simulink model "Overtaking_Integrated"  (R2020b)
settings: Solver=ode23tb  StartTime=0.0  StopTime=25  FixedStep=.01  RelTol=5e-3  EnableMultiTasking=on
InitFcn:
  | %SimulationParameters;
StartFcn:
  | %tic
StopFcn:
  | %toc
  | save(['SimOutputs\' char(datetime('now','Format','y_M_d_HH_mm_ss')) '_' 'sim_out.mat'], 'logsout');
model workspace (MAT data in the model file):
  DLCXref = [-3.2158 4.0142 4.2842 14.7842 29.7842 30.2842 41.7842 46.7842 56.7842]
  DLCYref = [-3.1012 -3.1012 -7.6012 -7.1012 -6.8512 -1.6012 -1.8512 -3.1012 -3.1012]
  Downshift_Speeds = [9.5625  23.0625  36.5625  47.8125  59.0625  68.90625  78.75; 12.9375  26.4375  39.9375  51.1875  62.4375  72.84375  83.25; 16.3125  29.8125  43.3125  54.5625  65.8125  76.78125  87.75; 19.6875  33.1875  46.6875  57.9375  69.1875  80.71875  92.25]
  EngRevLim = 7000
  Pedal_Positions = [0.1 0.4 0.5 0.9]
  Upshift_Speeds = [12.9375  26.4375  39.9375  51.1875  62.4375  72.84375  83.25; 16.3125  29.8125  43.3125  54.5625  65.8125  76.78125  87.75; 19.6875  33.1875  46.6875  57.9375  69.1875  80.71875  92.25; 33  52.5  77.25  100.5  138.75  161.875  185]
  VEH.Mass = 1181
  VEH.StaticNormalFrontLoad.FR = 264.666666667
  VEH.StaticNormalFrontLoad.FL = 264.666666667
  VEH.StaticNormalRearLoad.RR = 322
  VEH.StaticNormalRearLoad.RL = 322
  VEH.WheelBase = 3.075
  VEH.FrontAxlePositionfromCG = 1.515
  VEH.RearAxlePositionfromCG = 1.504
  VEH.HeightCG = 0.134
  VEH.FrontalArea = 2.11
  VEH.DragCoefficient = 0.33
  VEH.NumberOfWheelsPerAxle = 2
  VEH.PitchMomentInertia = 1922.66666667
  VEH.RollMomentInertia = 432.333333333
  VEH.YawMomentInertia = 2066
  VEH.SteeringRatio = 18
  VEH.TrackWidth = 1.922
  VEH.SprungMass = 1096.72266667
  VEH.InitialLongPosition = 0
  VEH.InitialLatPosition = 2.9015
  VEH.InitialVertPosition = 0
  VEH.InitialRollAngle = 0
  VEH.InitialPitchAngle = 0
  VEH.InitialYawAngle = 0
  VEH.InitialLongVel = 0
  VEH.InitialLatVel = 0
  VEH.InitialVertVel = 0
  VEH.InitialRollRate = 0
  VEH.InitialPitchRate = 0
  VEH.InitialYawRate = 0
values from neighbouring files (symbols this model uses):
  abortTrigger = 0.0    [AOTDataDictionary.sldd]
  Dmax = 3.0    [AOTDataDictionary.sldd]
  dt = 0.05    [AOTDataDictionary.sldd]
  egoVehLength = 4.948    [AOTDataDictionary.sldd]
  egoVehWidth = 2.009    [AOTDataDictionary.sldd]
  gamma = 0.5    [AOTDataDictionary.sldd]
  inflationFactor = 1.1    [AOTDataDictionary.sldd]
  inflexPoint = 0.0    [AOTDataDictionary.sldd]
  L = 3.705    [AOTDataDictionary.sldd]
  npcVehLength = 4.848    [AOTDataDictionary.sldd]
  npcVehWidth = 1.842    [AOTDataDictionary.sldd]
  plotSampleTime = 0.1    [AOTDataDictionary.sldd]
  SenseResolution = 0.1    [AOTDataDictionary.sldd]
  XSenseRange = 20.0    [AOTDataDictionary.sldd]
  YSenseRange = 20.0    [AOTDataDictionary.sldd]
undefined symbols (not defined in the file or in its folder): driving
libraries: simulink x10, drivingscenarioandsensors x5, autolibutils x4, sim3dautolib x3, sim3dlib x2, autolibshared x1, vehdynlibdriver x1, vehdynlibscenariocommon x1, pid_lib x1, vehdynlibsens x1
(part 1 of 3)
settings Model: DataDictionary=AOTDataDictionary.sldd  ModifiedByFormat=The MathWorks, Inc.  OrderedModelArguments=off  Creator=The MathWorks, Inc.  LastModifiedBy=The MathWorks, Inc.
settings SolverCC: SolverJacobianMethodControl=FullPerturbation  ZeroCrossAlgorithm=Adaptive  AutoInsertRateTranBlk=on  InsertRTBMode=Never (minimum delay)  DecoupledContinuousIntegration=on  MinimalZcImpactIntegration=on
settings DataIOCC: ReturnWorkspaceOutputs=off
settings DebuggingCC: SignalInfNanChecking=error  ArtificialAlgebraicLoopMsg=none  MaskedZcDiagnostic=none  IgnoredZcDiagnostic=none  ModelReferenceExtraNoncontSigs=none  PregeneratedLibrarySubsystemCodeDiagnostic=none  ArithmeticOperatorsInVariantConditions=warning
settings ModelReferenceCC: UpdateModelReferenceTargets=IfOutOfDate  ModelReferenceMinAlgLoopOccurrences=on  PropagateSignalLabelsOutOfModel=off
settings SFSimCC: SimUseLocalCustomCode=off
settings RTWCC: RTWUseLocalCustomCode=off

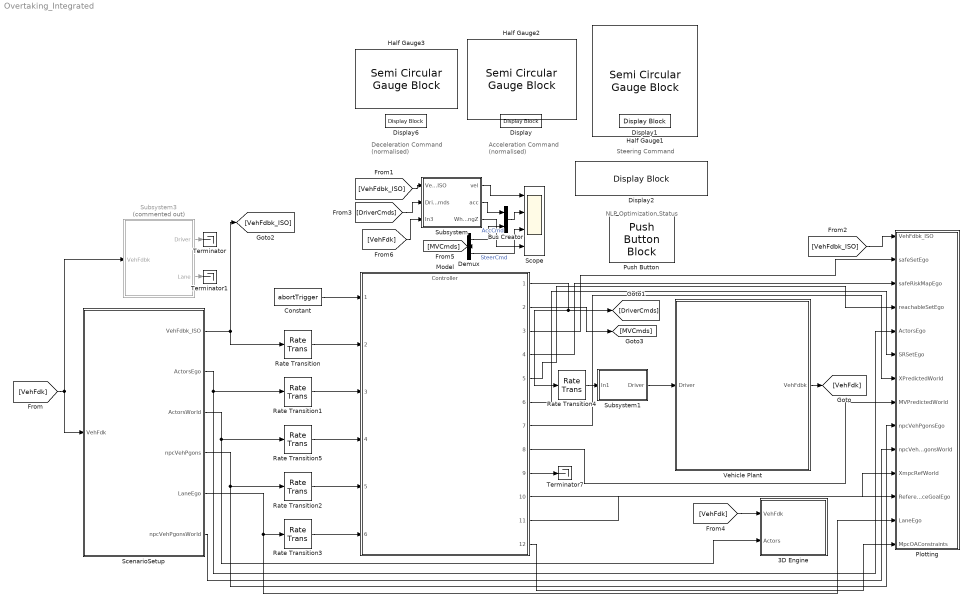
== system Overtaking_Integrated ==
  note: Deceleration Command
      | (normalised)
  note: NLP Optimization Status
  note: Acceleration Command
      | (normalised)
  note: Steering Command
  3D Engine : Subsystem  Variant=on  VariantControlMode=label  LabelModeActiveChoice=0  mask(3D Engine){engine3D=Disabled, SceneDesc=Straight road, dt3D=dt, defaultPos=User-specified, X_o=0, Y_o=2.9015, Z_o=0, phi_o=0, theta_o=0, psi_o=0}
      mask prompts: engine3D "3D Engine"; SceneDesc "Scene:"; dt3D "Engine frame rate, dt3D [s]:"; X_o "Initial longitudinal position, X_o [m]:"; Y_o "Initial lateral position, Y_o [m]:"; Z_o "Initial vertical position, Z_o [m]:"; phi_o "Initial roll angle, phi_o [rad]:"; theta_o "Initial pitch angle, theta_o [rad]:"; psi_o "Initial yaw angle, psi_o [rad]:"
      mask help: This subsystem contains the interface blocks which permit the display of the vehicle in the 3D virtual environment. Enable it to view the simulation progress, disable it to inhibit the display.
      mask init:
      | switch get_param(gcb,'engine3D')
      |     case 'Disabled'
      |         set_param(gcb,'OverrideUsingVariant','0')
      |         try
      |             set_param([bdroot '/Vehicle Plant/Environment/Ground Feedback'],'OverrideUsingVariant','0')
      |         catch
      |             disp('Warning: No ground feedback sensor not set')
      |         end
      |     case 'Enabled'
      |         set_param(gcb,'OverrideUsingVariant','1')
      |         try
      |             set_param([bdroot '/Vehicle Plant/Environment/Ground Feedback'],'OverrideUsingVariant','1')
      |         catch
      |             disp('Warning: No ground feedback sensor not set')
      |         end
      |     otherwise
      |         set_param(gcb,'OverrideUsingVariant','0')
      | end
      settings: AttributesFormatString=|
      | %<SceneDesc>
      | %<engine3D>
      mask Help: eval('vdynblkshelp(''vdynblks3dengine'')');
      mask TypeOptions engine3D: Enabled | Disabled
      mask Callback engine3D:
      | switch get_param(gcb,'engine3D')
      |     case 'Disabled'
      |         set_param(gcb,'OverrideUsingVariant','0')
      |     case 'Enabled'
      |        set_param(gcb,'OverrideUsingVariant','1')
      |     otherwise
      |        set_param(gcb,'OverrideUsingVariant','0')
      | end
      mask TypeOptions SceneDesc: 3D Engine/Simulation 3D Scene Configuration/SceneDesc
      mask Callback SceneDesc:
      | defaultStatus = get_param(gcb,'defaultPos');
      | if strcmp(defaultStatus,'Recommended for scene')
      | sceneType = get_param(gcb,'SceneDesc');
      | switch sceneType
      |     case 'Straight road'
      |         set_param(gcb,'X_o', '-118')
      |         set_param(gcb,'Y_o', '3.125')
      |         set_param(gcb,'Z_o', '0')
      |         set_param(gcb,'phi_o', '0')
      |         set_param(gcb,'theta_o', '0')
      |         set_param(gcb,'psi_o', '0')
      |     case 'Curved road'
      |         set_param(gcb,'X_o', '0.2')
      |         set_param(gcb,'Y_o', '-1605.0')
      |         set_param(gcb,'Z_o', '0')
      |         set_param(gcb,'phi_o', '0')
      |         set_param(gcb,'theta_o', '0')
      |         set_param(gcb,'psi_o', '-156*pi/180')
      |     case 'Parking lot'
      |         set_param(gcb,'X_o', '-104.0')
      |         set_param(gcb,'Y_o', '-9.7')
      |         set_param(gcb,'Z_o', '0')
      |         set_param(gcb,'phi_o', '0')
      |         set_param(gcb,'theta_o', '0')
      |         set_param(gcb,'psi_o', '0')
      |     case 'Double lane change'
      |         set_param(gcb,'X_o', '0')
      |         set_param(gcb,'Y_o', '3.125')
      |         set_param(gcb,'Z_o', '0')
      |         set_param(gcb,'phi_o', '0')
      |         set_param(gcb,'theta_o', '0')
      |         set_param(gcb,'psi_o', '0')
      |     case 'Open surface'
      |         set_param(gcb,'X_o', '0')
      |         set_param(gcb,'Y_o', '0')
      |         set_param(gcb,'Z_o', '0')
      |         set_param(gcb,'phi_o', '0')
      |         set_param(gcb,'theta_o', '0')
      |         set_param(gcb,'psi_o', '0')
      |     case 'US highway'
      |         set_param(gcb,'X_o', '3592.00')
      |         set_param(gcb,'Y_o', '2617.00')
      |         set_param(gcb,'Z_o', '-1.0')
      |         set_param(gcb,'phi_o', '0')
      |         set_param(gcb,'theta_o', '0')
      |         set_param(gcb,'psi_o', '0')
      |     case 'US city block'
      |         set_param(gcb,'X_o', '-125.19')
      |         set_param(gcb,'Y_o', '1.65')
      |         set_param(gcb,'Z_o', '-0.04')
      |         set_param(gcb,'phi_o', '0')
      |         set_param(gcb,'theta_o', '0')
      |         set_param(gcb,'psi_o', '0')
      |     case 'Large parking lot'
      |         set_param(gcb,'X_o', '45.0')
      |         set_param(gcb,'Y_o', '54.7')
      |         set_param(gcb,'Z_o', '0.0')
      |         set_param(gcb,'phi_o', '0')
      |         set_param(gcb,'theta_o', '0')
      |         set_param(gcb,'psi_o', '-pi/2')
      |     case 'Virtual Mcity'
      |         set_param(gcb,'X_o', '-26.0')
      |         set_param(gcb,'Y_o', '76.0')
      |         set_param(gcb,'Z_o', '0.0')
      |         set_param(gcb,'phi_o', '0')
      |         set_param(gcb,'theta_o', '0')
      |         set_param(gcb,'psi_o', '-40*pi/180')
      |     otherwise
      |         set_param(gcb,'X_o', '0')
      |         set_param(gcb,'Y_o', '0')
      |         set_param(gcb,'Z_o', '0')
      |         set_param(gcb,'phi_o', '0')
      |         set_param(gcb,'theta_o', '0')
      |         set_param(gcb,'psi_o', '0')
      | end
      | end
      mask TypeOptions defaultPos: Recommended for scene | User-specified
      mask DialogControl engineConfig Prompt: 3D Engine Settings
      mask DialogControl posSetup Prompt: Initial vehicle position
      mask DialogControl posSetupDesc Prompt: To use these initial vehicle positions, first Apply the initial values and then click Update the model workspaces with the initial values.
      mask DialogControl setModelPos Prompt: Update model workspaces with initial values
      mask DialogControl setModelPos Callback:
      | if strcmp(get_param(bdroot(gcb),'SimulationStatus'),'stopped')
      |     sceneType = get_param(gcb,'SceneDesc');
      |     rootModel = bdroot(gcb);
      |     ws = get_param(rootModel, 'modelworkspace');
      |     VEH = getVariable(ws,'VEH');
      |     ParamList={'X_o',[1,1],{};'Y_o',[1,1],{};'Z_o',[1,1],{};'phi_o',[1,1],{'gte',-pi/2;'lte',pi/2};'theta_o',[1,1],{'gte',-pi/2;'lte',pi/2};'psi_o',[1,1],{'gte',-2*pi;'lte',2*pi}};
      |     paramStruct = autoblkscheckparams(gcb, '3D Engine',ParamList);
      |     VEH.InitialLongPosition = paramStruct.X_o;
      |     VEH.InitialLatPosition = paramStruct.Y_o;
      |     VEH.InitialVertPosition = paramStruct.Z_o;
      |     VEH.InitialRollAngle = paramStruct.phi_o;
      |     VEH.InitialPitchAngle = paramStruct.theta_o;
      |     VEH.InitialYawAngle = paramStruct.psi_o;
      |     assignin(ws,'VEH',VEH);
      |     modelList = {'PassVeh14DOF','PassVeh7DOF'};
      |     for idx =1:length(modelList)
      | %         try
      |             load_system(modelList{idx});
      |             ws = get_param(modelList{idx}, 'modelworkspace');
      |             assignin(ws,'VEH',VEH);
      |             save_system(modelList{idx});
      |             close_system(modelList{idx});
      | %         catch
      | %             disp(['Cannot find ' modelList{idx}])
      | %         end
      |     end
      | end
      mask Display: disp('3D Engine')
  Bus Creator : BusCreator  Inputs=2
  Constant : Constant  Value=abortTrigger  OutDataTypeStr=boolean
  Demux : Demux  Outputs=2
  Display{,1..2,6} (4 alike) : DisplayBlock  LabelPosition=Hide  Format=short  Transparency=1
  Half Gauge1 : SemiCircularGaugeBlock  ScaleMin=-1.5  ScaleMax=1.5
  Half Gauge2 : SemiCircularGaugeBlock  ScaleMax=1
  Half Gauge3 : SemiCircularGaugeBlock  ScaleMax=1
  Model : ModelReference  ModelNameDialog=Controller.slx  SimulationMode=Normal  ModelReferenceVersion=1.287
  Plotting : Subsystem  TreatAsAtomicUnit=on  SystemSampleTime=plotSampleTime
  Push Button : PushButtonBlock  LabelPosition=Bottom
  Rate Transition{,1..5} (6 alike) : RateTransition
  ScenarioSetup : Subsystem
  Scope : Scope  NumInputPorts=4
  Subsystem : Subsystem
  Subsystem1 : Subsystem
  Subsystem3 : Subsystem  Commented=on
  Terminator : Terminator
  Terminator1 : Terminator
  Terminator7 : Terminator
  Vehicle Plant : Subsystem
  wires:
  Model/1 -> Rate Transition4/1, [DriverCmds]
  Rate Transition/1 -> Model/2
  Rate Transition2/1 -> Model/5
  Rate Transition3/1 -> Model/6
  Rate Transition1/1 -> Model/3
  Model/9 -> Terminator7/1
  Rate Transition4/1 -> Subsystem1/1(In1)
  [VehFdbk_ISO] -> Subsystem/1(VehFdbk_ISO)
  [DriverCmds] -> Subsystem/2(DriverCmds)
  Subsystem1/1(Driver) -> Vehicle Plant/1(Driver)
  ScenarioSetup/1(VehFdbk_ISO) -> [VehFdbk_ISO], Rate Transition/1
  ScenarioSetup/4(npcVehPgons) -> Plotting/9(npcVehPgonsEgo), Rate Transition2/1
  ScenarioSetup/5(LaneEgo) -> Plotting/13(LaneEgo), Rate Transition3/1
  ScenarioSetup/2(ActorsEgo) -> Rate Transition1/1, Plotting/5(ActorsEgo)
  Subsystem3/1(Driver) -> Terminator/1
  [VehFdbk_ISO] -> Plotting/1(VehFdbk_ISO)
  Model/3 -> Plotting/2(safeSetEgo)
  Model/4 -> Plotting/3(safeRiskMapEgo)
  Model/5 -> Plotting/4(reachableSetEgo)
  Model/6 -> Plotting/6(SRSetEgo)
  Model/7 -> Plotting/7(XPredictedWorld)
  Model/8 -> Plotting/8(MVPredictedWorld)
  Model/10 -> Plotting/11(XmpcRefWorld)
  Model/11 -> Plotting/12(ReferenceGoalEgo)
  Model/12 -> Plotting/14(MpcOAConstraints)
  [VehFdk] -> Subsystem3/1(VehFdbk), ScenarioSetup/1(VehFdk)
  ScenarioSetup/3(ActorsWorld) -> 3D Engine/2(Actors), Rate Transition5/1
  [VehFdk] -> 3D Engine/1(VehFdk)
  Subsystem3/2(Lane) -> Terminator1/1
  Subsystem/1(vel) -> Scope/1
  Subsystem/2(acc) -> Bus Creator/1
  Model/2 -> [MVCmds]
  [MVCmds] -> Demux/1
  Demux/1 -> Bus Creator/2  "AccCmd"
  Demux/2 -> Scope/3  "SteerCmd"
  Bus Creator/1 -> Scope/2
  ScenarioSetup/6(npcVehPgonsWorld) -> Plotting/10(npcVehPgonsWorld)
  Rate Transition5/1 -> Model/4
  Vehicle Plant/1(VehFdbk) -> [VehFdk]
  [VehFdk] -> Subsystem/3(In3)
  Subsystem/3(WheelAngZ) -> Scope/4
  Constant/1 -> Model/1

== system Overtaking_Integrated/3D Engine ==
  note: 1) Add Subsystem or Model blocks as valid variant choices.
      | 2) You cannot connect blocks at this level. At simulation, connectivity is automatically
      | determined, based on the active variant and port name matching.
  VehFdk : Inport
  Actors : Inport  Port=2
  3D Engine : Subsystem  VariantControl=1
  3D Engine Disabled : Subsystem  VariantControl=0

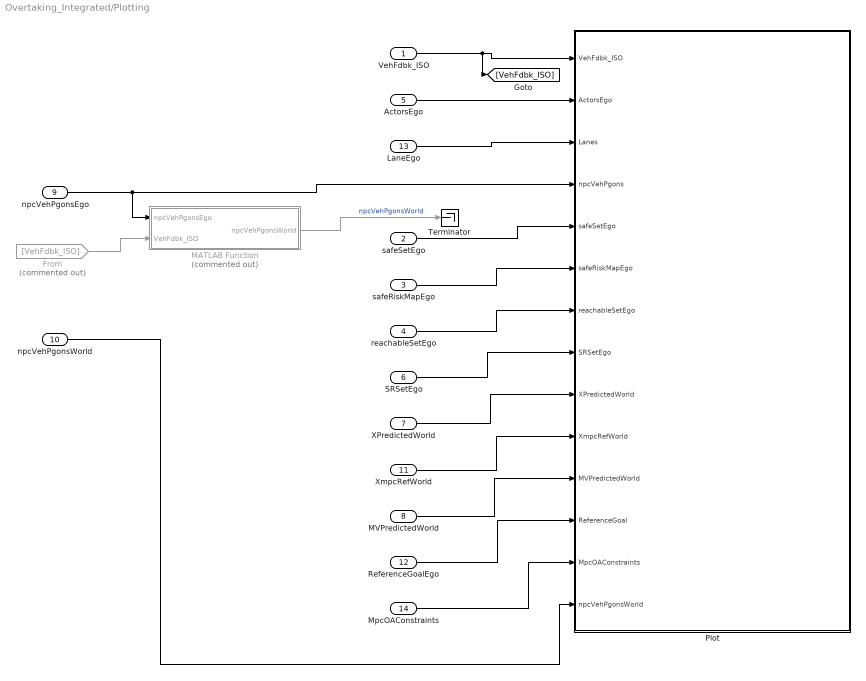
== system Overtaking_Integrated/Plotting ==
  VehFdbk_ISO : Inport
  safeSetEgo : Inport  Port=2
  safeRiskMapEgo : Inport  Port=3
  reachableSetEgo : Inport  Port=4
  ActorsEgo : Inport  Port=5
  SRSetEgo : Inport  Port=6
  XPredictedWorld : Inport  Port=7
  MVPredictedWorld : Inport  Port=8
  npcVehPgonsEgo : Inport  Port=9
  npcVehPgonsWorld : Inport  Port=10
  XmpcRefWorld : Inport  Port=11
  ReferenceGoalEgo : Inport  Port=12
  LaneEgo : Inport  Port=13
  MpcOAConstraints : Inport  Port=14
  From : From  Commented=on  GotoTag=VehFdbk_ISO
  MATLAB Function : MATLAB Function  Commented=on  TreatAsAtomicUnit=on
  Plot : MATLAB Function  TreatAsAtomicUnit=on  SystemSampleTime=plotSampleTime
  Terminator : Terminator
  wires:
  SRSetEgo/1 -> Plot/8(SRSetEgo)
  safeRiskMapEgo/1 -> Plot/6(safeRiskMapEgo)
  npcVehPgonsEgo/1 -> MATLAB Function/1(npcVehPgonsEgo), Plot/4(npcVehPgons)
  VehFdbk_ISO/1 -> [VehFdbk_ISO], Plot/1(VehFdbk_ISO)
  MVPredictedWorld/1 -> Plot/11(MVPredictedWorld)
  XPredictedWorld/1 -> Plot/9(XPredictedWorld)
  ActorsEgo/1 -> Plot/2(ActorsEgo)
  LaneEgo/1 -> Plot/3(Lanes)
  reachableSetEgo/1 -> Plot/7(reachableSetEgo)
  safeSetEgo/1 -> Plot/5(safeSetEgo)
  XmpcRefWorld/1 -> Plot/10(XmpcRefWorld)
  ReferenceGoalEgo/1 -> Plot/12(ReferenceGoal)
  MpcOAConstraints/1 -> Plot/13(MpcOAConstraints)
  From/1 -> MATLAB Function/2(VehFdbk_ISO)
  MATLAB Function/1(npcVehPgonsWorld) -> Terminator/1  "npcVehPgonsWorld"
  npcVehPgonsWorld/1 -> Plot/14(npcVehPgonsWorld)

== system Overtaking_Integrated/ScenarioSetup ==
  VehFdk : Inport
  GenerateNPCPolygons : Subsystem
  Scenario Reader : Subsystem
  VehFdbk_ISO : Outport
  ActorsEgo : Outport  Port=2
  ActorsWorld : Outport  Port=3
  npcVehPgons : Outport  Port=4
  LaneEgo : Outport  Port=5
  npcVehPgonsWorld : Outport  Port=6
  wires:
  Scenario Reader/1(VehFdbk_ISO) -> GenerateNPCPolygons/2(VehFdbk_ISO), VehFdbk_ISO/1  "VehFdbk_ISO"
  Scenario Reader/2(ActorsEgo) -> GenerateNPCPolygons/1(ActorsEgo), ActorsEgo/1  "ActorsEgo"
  GenerateNPCPolygons/1(npcVehPgons) -> npcVehPgons/1  "npcVehPgons"
  Scenario Reader/4(LaneEgo) -> LaneEgo/1  "LaneEgo"
  VehFdk/1 -> Scenario Reader/1(VehFdk)
  Scenario Reader/3(ActorsWorld) -> ActorsWorld/1  "ActorsWorld"
  GenerateNPCPolygons/2(npcVehPgonsWorld) -> npcVehPgonsWorld/1

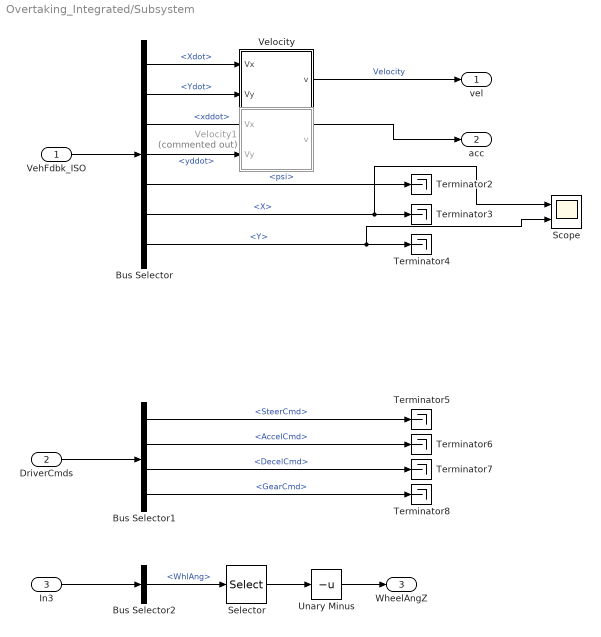
== system Overtaking_Integrated/Subsystem ==
  VehFdbk_ISO : Inport
  DriverCmds : Inport  Port=2
  In3 : Inport  Port=3
  Bus Selector : BusSelector  OutputSignals=Velocity.Xdot,Velocity.Ydot,Acceleration.xddot,Acceleration.yddot,Orientation.psi,Position.X,Position.Y
  Bus Selector1 : BusSelector  OutputSignals=SteerCmd,AccelCmd,DecelCmd,GearCmd
  Bus Selector2 : BusSelector  OutputSignals=Wheels.Steering.WhlAng
  Scope : Scope  NumInputPorts=2
  Selector : Selector  InputPortWidth=4  IndexOptions=Index vector (dialog)  Indices=[1]  OutputSizes=1
  Terminator{2..8} (7 alike) : Terminator
  Unary Minus : UnaryMinus
  Velocity : Subsystem
  Velocity1 : Subsystem  Commented=on
  vel : Outport
  acc : Outport  Port=2  Unit=m/s^2
  WheelAngZ : Outport  Port=3
  wires:
  Bus Selector/2 -> Velocity/2(Vy)  "<Ydot>"
  Bus Selector/1 -> Velocity/1(Vx)  "<Xdot>"
  VehFdbk_ISO/1 -> Bus Selector/1
  Velocity/1(v) -> vel/1  "Velocity"
  Bus Selector/3 -> acc/1  "<xddot>"
  Bus Selector/4 -> Velocity1/2(Vy)  "<yddot>"
  Bus Selector/5 -> Terminator2/1  "<psi>"
  Bus Selector/6 -> Scope/1, Terminator3/1  "<X>"
  Bus Selector/7 -> Scope/2, Terminator4/1  "<Y>"
  DriverCmds/1 -> Bus Selector1/1
  Bus Selector1/1 -> Terminator5/1  "<SteerCmd>"
  Bus Selector1/4 -> Terminator8/1  "<GearCmd>"
  Bus Selector1/3 -> Terminator7/1  "<DecelCmd>"
  Bus Selector1/2 -> Terminator6/1  "<AccelCmd>"
  In3/1 -> Bus Selector2/1
  Bus Selector2/1 -> Selector/1  "<WhlAng>"
  Selector/1 -> Unary Minus/1
  Unary Minus/1 -> WheelAngZ/1

== system Overtaking_Integrated/Subsystem1 ==
  In1 : Inport
  Bus Creator : BusCreator  Inputs=4  OutDataTypeStr=Bus: DriverCmd  NonVirtualBus=on
      settings: InheritFromInputs=off
  Bus Selector : BusSelector  OutputSignals=SteerCmd,AccelCmd,DecelCmd,GearCmd
  Unary Minus : UnaryMinus
  Driver : Outport
  wires:
  In1/1 -> Bus Selector/1
  Bus Selector/1 -> Unary Minus/1  "<SteerCmd>"
  Unary Minus/1 -> Bus Creator/1
  Bus Selector/2 -> Bus Creator/2  "<AccelCmd>"
  Bus Selector/3 -> Bus Creator/3  "<DecelCmd>"
  Bus Selector/4 -> Bus Creator/4  "<GearCmd>"
  Bus Creator/1 -> Driver/1

== system Overtaking_Integrated/Subsystem3 ==
  VehFdbk : Inport
  Driver Commands : Subsystem  VariantControl=0  mask{driverType=Predictive Driver}
      mask prompts: driverType "Vehicle command mode"
      mask init:
      | [~]=vdynblksdrvrconfig(gcb)
      settings: AttributesFormatString=%<driverType>
      mask Help: eval('vdynblkshelp(''vdcrdriver'')');
      mask TypeOptions driverType: Longitudinal Driver | Predictive Driver | Open Loop
      mask Display: image('driverlatlong.png');
  Lane Change Reference Generator : vehdynlibscenariocommon/Lane Change Reference Generator  ssMode=Initialize from model  ssVar=dlcSS35mph  t_start=1  XGate=175  xdot_r=35  xdotUnit=mph  xStart=2  vehW=2  latoff=VEH.InitialLatPosition  lattoff=VEH.InitialLatPosition  centerSwitch=off  xSimStop=off  latRefbp=DLCXref  latRef=DLCYref  X_o=175  Y_o=VEH.InitialLatPosition  psi_o=VEH.InitialYawAngle  ssTol=1  ssMaxTime=30  ssWSName=dlcSS35mph  aMode=2
      link override ISO 3888-2/Lateral Reference: LabelModeActiveChoice=0
      settings: SourceProductBaseCode=VE
  Driver : Outport
  Lane : Outport  Port=2
  wires:
  Lane Change Reference Generator/2 -> Driver Commands/1(VehRef)
  Driver Commands/1(Driver) -> Driver/1
  Lane Change Reference Generator/1 -> Lane/1
  VehFdbk/1 -> Lane Change Reference Generator/1, Driver Commands/2(VehFdbk)

== system Overtaking_Integrated/Vehicle Plant ==
  Driver : Inport
  Controllers : Subsystem
      mask Display: image('SystemControllers.png')
  Environment : Subsystem
      mask Display: disp('Environment')
  Passenger Vehicle : Subsystem
      mask Display: image('PassengerVehicle.png')
  Sensors : Subsystem
      mask Display: image('sensorimu.png'); % Use "Edit Image" on toolstrip to change.
  VehFdbk : Outport
  wires:
  Controllers/1(CntrlTx) -> Passenger Vehicle/2(Cntrl), Sensors/3(CntrlTx)
  Driver/1 -> Passenger Vehicle/1(Driver)
  Environment/1(Env) -> Passenger Vehicle/3(Env), Sensors/2(Env)
  Passenger Vehicle/1(VehFdbk) -> VehFdbk/1, Sensors/1(VehFdbk)
  Sensors/1(CntrlRx) -> Controllers/1(CntrlRx)

== system Overtaking_Integrated/3D Engine/3D Engine ==
  VehFdk : Inport
  Actors : Inport  Port=2
  Cuboid To 3D Simulation : drivingscenarioandsensors/Cuboid To 3D Simulation  SpecifyActorID=on  ActorIDToConvert=2  SimulateUsing=Interpreted execution
      settings: SourceProductBaseCode=DR
  Cuboid To 3D Simulation1 : drivingscenarioandsensors/Cuboid To 3D Simulation  SpecifyActorID=on  ActorIDToConvert=3  SimulateUsing=Interpreted execution
      settings: SourceProductBaseCode=DR
  Generate Translation Rotation : Subsystem
  Scale : Subsystem
  Simulation 3D Scene Configuration : sim3dlib/Simulation 3D Scene Configuration  Priority=0  ProjectFormat=Default Scenes  SceneDesc=Straight road  ProjectName=L:\Bvehicle\matlab\toolbox\shared\sim3d_projects\automotive_project\UE4\WindowsNoEditor\VehicleSimulation.exe  ScenePath=/Game/Maps/HwStrght  vehTagList={'EgoVehicle';'LeadVehicle1';'LeadVehicle2';'Scene Origin'}  vehTag=EgoVehicle  OpVisEn=off  Ts=dt3D  EnableWindow=on  sensorTag=MainCamera1  sensorId=1  sensorName=MainCamera1  mountLoc=Origin  offsetFlag=off  tmountOffset=[0, 0, 0]  rmountOffset=[0, 0, 0]  HorizontalResolution=1280  VerticalResolution=720  HorizontalFOV=60  mountPoint=[0 0 0]  mountOrientation=[0 0 0]  aMode=aMode  ID=1
      settings: SourceProductBaseCode=DR,UV,VE
  Simulation 3D Vehicle : sim3dautolib/Simulation 3D Vehicle  Priority=-1  PassVehMesh=Muscle car  VehColor=Red  ActorName=EgoVehicle  Translation=[VEH.InitialLongPosition VEH.InitialLatPosition -VEH.InitialVertPosition; 0 0 0; 0 0 0; 0 0 0; 0 0 0]  Rotation=[VEH.InitialRollAngle VEH.InitialPitchAngle VEH.InitialYawAngle; 0 0 0; 0 0 0; 0 0 0; 0 0 0]  Scale=ones( 5, 3 )  SampleTime=dt3D  ActorType=SimulinkVehicle  ID=C  aMode=2  ActorTag=EgoVehicle
      settings: SourceProductBaseCode=DR,UV,VE
  Vehicle in Adjacent Lane : sim3dautolib/Simulation 3D Vehicle with Ground Following  Priority=-1  PassVehMesh=Sedan  VehColor=Orange  InitialPos=[0, -3, 0]  InitialRot=[0, 0, 0]  ActorName=LeadVehicle1  SampleTime=dt3D  ActorType=SimulinkVehicle  ID=C  aMode=3  ActorTag=LeadVehicle1  CoordinateScheme=ISO  TransformOutportEnabled=off
      settings: SourceProductBaseCode=DR,UV,VE
  Vehicle in Adjacent Lane1 : sim3dautolib/Simulation 3D Vehicle with Ground Following  Priority=-1  PassVehMesh=Sedan  VehColor=Orange  InitialPos=[0, -3, 0]  InitialRot=[0, 0, 0]  ActorName=LeadVehicle2  SampleTime=dt3D  ActorType=SimulinkVehicle  ID=C  aMode=3  ActorTag=LeadVehicle2  CoordinateScheme=ISO  TransformOutportEnabled=off
      settings: SourceProductBaseCode=DR,UV,VE
  wires:
  Scale/1(ScaleOut) -> Simulation 3D Vehicle/3
  Generate Translation Rotation/2(VehRotation) -> Simulation 3D Vehicle/2
  Generate Translation Rotation/1(VehTranslation) -> Simulation 3D Vehicle/1
  Cuboid To 3D Simulation/1 -> Vehicle in Adjacent Lane/1
  Cuboid To 3D Simulation/3 -> Vehicle in Adjacent Lane/3
  Cuboid To 3D Simulation/2 -> Vehicle in Adjacent Lane/2
  Actors/1 -> Cuboid To 3D Simulation1/1, Cuboid To 3D Simulation/1
  VehFdk/1 -> Generate Translation Rotation/1(VehFdk)
  Cuboid To 3D Simulation1/2 -> Vehicle in Adjacent Lane1/2
  Cuboid To 3D Simulation1/3 -> Vehicle in Adjacent Lane1/3
  Cuboid To 3D Simulation1/1 -> Vehicle in Adjacent Lane1/1

== system Overtaking_Integrated/3D Engine/3D Engine Disabled ==
  VehFdk : Inport
  Actors : Inport  Port=2
  Terminator : Terminator
  Terminator1 : Terminator
  wires:
  VehFdk/1 -> Terminator/1
  Actors/1 -> Terminator1/1

== system Overtaking_Integrated/ScenarioSetup/GenerateNPCPolygons ==
  ActorsEgo : Inport
  VehFdbk_ISO : Inport  Port=2
  GenerateObstaclepolygons : MATLAB Function  TreatAsAtomicUnit=on
  GenerateObstaclepolygons1 : MATLAB Function  Commented=on  TreatAsAtomicUnit=on
  Ground : Ground
  npcVehPgons : Outport
  npcVehPgonsWorld : Outport  Port=2
  wires:
  GenerateObstaclepolygons/1(npcVehPgons) -> npcVehPgons/1  "npcVehiclePolygons"
  ActorsEgo/1 -> GenerateObstaclepolygons/1(ActorsEgo)
  VehFdbk_ISO/1 -> GenerateObstaclepolygons/2(VehFdbk_ISO)
  Ground/1 -> npcVehPgonsWorld/1

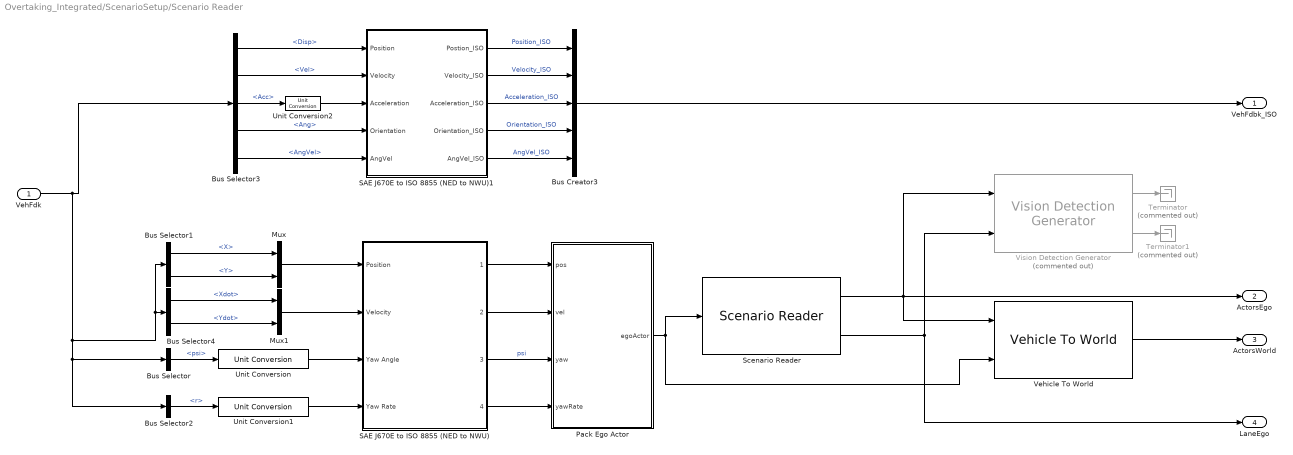
== system Overtaking_Integrated/ScenarioSetup/Scenario Reader ==
  VehFdk : Inport
  Bus Creator3 : BusCreator  Inputs=5  OutDataTypeStr=Bus: Veh_Fdbk  NonVirtualBus=on
      settings: InheritFromInputs=off
  Bus Selector : BusSelector  OutputSignals=Body.InertFrm.Cg.Ang.psi
  Bus Selector1 : BusSelector  OutputSignals=Body.InertFrm.Cg.Disp.X,Body.InertFrm.Cg.Disp.Y
  Bus Selector2 : BusSelector  OutputSignals=Body.BdyFrm.Cg.AngVel.r
  Bus Selector3 : BusSelector  OutputSignals=Body.InertFrm.Cg.Disp,Body.InertFrm.Cg.Vel,Body.BdyFrm.Cg.Acc,Body.InertFrm.Cg.Ang,Body.BdyFrm.Cg.AngVel
  Bus Selector4 : BusSelector  OutputSignals=Body.InertFrm.Cg.Vel.Xdot,Body.InertFrm.Cg.Vel.Ydot
  Mux : Mux  Inputs=2
  Mux1 : Mux  Inputs=2
  Pack Ego Actor : MATLAB Function  TreatAsAtomicUnit=on
  SAE J670E to ISO 8855 (NED to NWU) : Subsystem
  SAE J670E to ISO 8855 (NED to NWU)1 : Subsystem
  Scenario Reader : drivingscenarioandsensors/Scenario Reader  ScenarioSource=From file  ScenarioFileName=D:\Projects\AutonomousOvertaking\AutonomousOvertaking\main\Scenario_definitions\Overtaking_Scenario_ConstantLVVelocity.mat  ScenarioVariableName=scenario  OutputCoordinateSystem=Vehicle coordinates  EgoVehicleSource=Input port  EgoVehicleActorID=1  OrientVehiclesOnRoad=off  OutputEgoVehiclePose=off  SampleTime=dt  LaneBoundaryOutput=All lane boundaries  LaneBoundaryDistance=-XSenseRange:SenseResolution:XSenseRange  LaneBoundaryLocation=Center of lane markings  BusNameSource=Property  BusName=BusActors  BusName2Source=Property  BusName2=BusLaneBoundaries  BusName3Source=Auto  BusName3=BusEgoActor  ShowCoordinateLabels=on  SimulateUsing=Interpreted execution
  Terminator : Terminator  Commented=on
  Terminator1 : Terminator  Commented=on
  Unit Conversion : UnitConversion  OutputType=Inherit: Inherit via back propagation
  Unit Conversion1 : UnitConversion  OutputType=Inherit: Inherit via back propagation
  Unit Conversion2 : UnitConversion  OutputType=Inherit: Inherit via back propagation
  Vehicle To World : drivingscenarioandsensors/Vehicle To World  BusNameSource=Property  BusName=BusVehicleToWorldActors  SimulateUsing=Interpreted execution
      settings: SourceProductBaseCode=DR
  Vision Detection Generator : drivingscenarioandsensors/Vision Detection Generator  Commented=on  SensorIndex=1  DetectorOutput=Lanes and objects  UpdateInterval=0.1  LaneUpdateInterval=0.1  SensorLocation=[ 1.9, 0 ]  Height=1.1  Yaw=0  Pitch=1  Roll=0  BusNameSource=Property  BusName=BusObjectDetections  BusName2Source=Property  BusName2=BusLaneDetections  MaxNumDetectionsSource=Property  MaxNumDetections=50  MaxNumLanesSource=Property  MaxNumLanes=30  DetectionCoordinates=Ego Cartesian  SimulateUsing=Interpreted execution  MaxRange=150  BoundingBoxAccuracy=5  ProcessNoiseIntensity=5  MaxSpeed=100  MaxAllowedOcclusion=0.5  MinObjectImageSize=[ 15, 15 ]  DetectionProbability=0.9  FalsePositivesPerImage=0.1  MinLaneImageSize=[ 20, 3 ]  LaneBoundaryAccuracy=3  HasNoise=on  InitialSeedSource=Repeatable  InitialSeed=0  UsedSeed=driving.internal.SimulinkUtilities.seedManager(gcb)  ActorProfilesSource=Parameters  ActorProfilesParameters=driving.internal.ActorProfilesParameters  ActorProfilesExpression=struct( 'ClassID', 0, 'Length', 4.7, 'Width', 1.8, 'Height', 1.4, 'OriginOffset', [ -1.35, 0, 0 ] )  Intrinsics=driving.internal.cameraIntrinsics
  VehFdbk_ISO : Outport
  ActorsEgo : Outport  Port=2
  ActorsWorld : Outport  Port=3
  LaneEgo : Outport  Port=4
  wires:
  Vehicle To World/1 -> ActorsWorld/1
  Scenario Reader/1 -> ActorsEgo/1, Vehicle To World/1, Vision Detection Generator/1
  Pack Ego Actor/1(egoActor) -> Scenario Reader/1, Vehicle To World/2
  Scenario Reader/2 -> LaneEgo/1, Vision Detection Generator/2
  Unit Conversion1/1 -> SAE J670E to ISO 8855 (NED to NWU)/4(Yaw Rate)
  Mux1/1 -> SAE J670E to ISO 8855 (NED to NWU)/2(Velocity)
  Bus Selector1/2 -> Mux/2  "<Y>"
  Unit Conversion/1 -> SAE J670E to ISO 8855 (NED to NWU)/3(Yaw Angle)
  Mux/1 -> SAE J670E to ISO 8855 (NED to NWU)/1(Position)
  Bus Selector1/1 -> Mux/1  "<X>"
  VehFdk/1 -> Bus Selector3/1, Bus Selector2/1, Bus Selector/1, Bus Selector4/1, Bus Selector1/1
  Bus Selector4/1 -> Mux1/1  "<Xdot>"
  Bus Selector4/2 -> Mux1/2  "<Ydot>"
  Bus Selector/1 -> Unit Conversion/1  "<psi>"
  Bus Selector2/1 -> Unit Conversion1/1  "<r>"
  SAE J670E to ISO 8855 (NED to NWU)/1(1) -> Pack Ego Actor/1(pos)
  SAE J670E to ISO 8855 (NED to NWU)/2(2) -> Pack Ego Actor/2(vel)
  SAE J670E to ISO 8855 (NED to NWU)/3(3) -> Pack Ego Actor/3(yaw)  "psi"
  SAE J670E to ISO 8855 (NED to NWU)/4(4) -> Pack Ego Actor/4(yawRate)
  Bus Selector3/1 -> SAE J670E to ISO 8855 (NED to NWU)1/1(Position)  "<Disp>"
  Bus Selector3/2 -> SAE J670E to ISO 8855 (NED to NWU)1/2(Velocity)  "<Vel>"
  Bus Selector3/4 -> SAE J670E to ISO 8855 (NED to NWU)1/4(Orientation)  "<Ang>"
  Bus Selector3/3 -> Unit Conversion2/1  "<Acc>"
  Bus Selector3/5 -> SAE J670E to ISO 8855 (NED to NWU)1/5(AngVel)  "<AngVel>"
  SAE J670E to ISO 8855 (NED to NWU)1/1(Postion_ISO) -> Bus Creator3/1  "Position_ISO"
  SAE J670E to ISO 8855 (NED to NWU)1/2(Velocity_ISO) -> Bus Creator3/2  "Velocity_ISO"
  SAE J670E to ISO 8855 (NED to NWU)1/3(Acceleration_ISO) -> Bus Creator3/3  "Acceleration_ISO"
  SAE J670E to ISO 8855 (NED to NWU)1/4(Orientation_ISO) -> Bus Creator3/4  "Orientation_ISO"
  SAE J670E to ISO 8855 (NED to NWU)1/5(AngVel_ISO) -> Bus Creator3/5  "AngVel_ISO"
  Bus Creator3/1 -> VehFdbk_ISO/1
  Vision Detection Generator/1 -> Terminator/1
  Vision Detection Generator/2 -> Terminator1/1
  Unit Conversion2/1 -> SAE J670E to ISO 8855 (NED to NWU)1/3(Acceleration)

== system Overtaking_Integrated/Subsystem/Velocity ==
  Vx : Inport
  Vy : Inport  Port=2
  Add : Sum
  Sqrt : Sqrt  SaturateOnIntegerOverflow=on
  Square : Math  Operator=square  SaturateOnIntegerOverflow=on
  Square1 : Math  Operator=square  SaturateOnIntegerOverflow=on
  v : Outport  Unit=m/s
  wires:
  Vy/1 -> Square1/1
  Vx/1 -> Square/1
  Sqrt/1 -> v/1
  Square1/1 -> Add/2
  Add/1 -> Sqrt/1
  Square/1 -> Add/1

== system Overtaking_Integrated/Subsystem/Velocity1 ==
  Vx : Inport
  Vy : Inport  Port=2
  Add : Sum
  Sqrt : Sqrt  SaturateOnIntegerOverflow=on
  Square : Math  Operator=square  SaturateOnIntegerOverflow=on
  Square1 : Math  Operator=square  SaturateOnIntegerOverflow=on
  v : Outport
  wires:
  Square/1 -> Add/1
  Add/1 -> Sqrt/1
  Square1/1 -> Add/2
  Sqrt/1 -> v/1
  Vx/1 -> Square/1
  Vy/1 -> Square1/1

== system Overtaking_Integrated/Subsystem3/Driver Commands ==
  VehRef : Inport
  VehFdbk : Inport  Port=2
  AccelGround : Ground
  BrakeGround : Ground
  Driver Commands : Subsystem  Variant=on  VariantControlMode=label  VariantControl=Variant1  LabelModeActiveChoice=1  AllowZeroVariantControls=on
  GearGround : Ground
  SteerGround : Ground
  Driver : Outport  VectorParamsAs1DForOutWhenUnconnected=off
  wires:
  VehRef/1 -> Driver Commands/1(VehRef)
  VehFdbk/1 -> Driver Commands/2(VehFdbk)
  Driver Commands/1(" Driver") -> Driver/1
  SteerGround/1 -> Driver Commands/3(SteerCmd)
  AccelGround/1 -> Driver Commands/4(Accel)
  BrakeGround/1 -> Driver Commands/5(Brake)
  GearGround/1 -> Driver Commands/6(Gear)

== system Overtaking_Integrated/Vehicle Plant/Controllers ==
  CntrlRx : Inport
  Active Differential Control : Subsystem  Variant=on  VariantControlMode=label  LabelModeActiveChoice=0
  Brake Controller : Subsystem
  Bus Creator{,1..2,4} (4 alike) : BusCreator  Inputs=1
  Bus Creator3 : BusCreator  Inputs=4
  Bus Selector : BusSelector  OutputSignals=Driver.DecelFdbk,Wheels.Omega,Wheels.Kappa
  Bus Selector1 : BusSelector  OutputSignals=Driver.AccFdbk,Driver.DecelFdbk,Driver.GearFdbk,Engine.EngSpd,Wheels.Omega
  Bus Selector2 : BusSelector  OutputSignals=Driver.AccFdbk,Engine.EngSpd
  Bus Selector3 : BusSelector  OutputSignals=Driver.AccFdbk,Driver.DecelFdbk,Driver.SteerFdbk,Driver.GearFdbk,Wheels.Omega,IMU.Acc,IMU.pqr
  ECU : Subsystem  SystemSampleTime=.01
  Ground : Ground
  Transmission Controller : Subsystem  Variant=on  VariantControlMode=label  VariantControl=Variant1  LabelModeActiveChoice=3
  CntrlTx : Outport  VectorParamsAs1DForOutWhenUnconnected=off
  wires:
  Bus Selector/3 -> Brake Controller/3(kappa)  "<Kappa>"
  Brake Controller/1(BrkPrsCmd) -> Bus Creator2/1  "BrkPrsCmd"
  Bus Selector/2 -> Brake Controller/2(Omega)  "<Omega>"
  CntrlRx/1 -> Bus Selector2/1, Bus Selector1/1, Bus Selector3/1, Bus Selector/1
  Bus Selector2/1 -> ECU/2(<Accel>)  "<AccFdbk>"
  Bus Creator/1 -> Bus Creator3/1  "ECU"
  Bus Creator1/1 -> Bus Creator3/2  "Transmission"
  Bus Creator2/1 -> Bus Creator3/3  "Brake"
  Bus Creator3/1 -> CntrlTx/1  "CntrlTx"
  Bus Creator4/1 -> Bus Creator3/4  "Diff"
  Active Differential Control/1(DiffPrsCmd) -> Bus Creator4/1  "DiffPrsCmd"
  Active Differential Control/2(TrqCmd) -> [DiffTrqCmd]
  ECU/1(EngTrqCmd) -> Bus Creator/1  "EngTrqCmd"
  Transmission Controller/1(" Gear") -> Bus Creator1/1  "GearCmd"
  [DiffTrqCmd] -> ECU/1(DiffTrqCmd)  "DiffTrqCmd"
  Ground/1 -> Transmission Controller/6(UpReq), Transmission Controller/7(DownReq)
  Bus Selector2/2 -> ECU/3(EngSpd)  "<EngSpd>"
  Bus Selector/1 -> Brake Controller/1(BrkCmd)  "<DecelFdbk>"
  Bus Selector1/5 -> Transmission Controller/5(Omega)  "<Omega>"
  Bus Selector1/2 -> Transmission Controller/2(BrkCmd)  "<DecelFdbk>"
  Bus Selector1/3 -> Transmission Controller/3(GearReq)  "<GearFdbk>"
  Bus Selector1/4 -> Transmission Controller/4(EngSpd)  "<EngSpd>"
  Bus Selector1/1 -> Transmission Controller/1(Accel)  "<AccFdbk>"
  Bus Selector3/1 -> Active Differential Control/1(Accel)  "<AccFdbk>"
  Bus Selector3/2 -> Active Differential Control/2(BrkCmd)  "<DecelFdbk>"
  Bus Selector3/3 -> Active Differential Control/3(Steer)  "<SteerFdbk>"
  Bus Selector3/4 -> Active Differential Control/4(GearFdbk)  "<GearFdbk>"
  Bus Selector3/5 -> Active Differential Control/5(Omega)  "<Omega>"
  Bus Selector3/6 -> Active Differential Control/6(axayaz)  "<Acc>"
  Bus Selector3/7 -> Active Differential Control/7(pqr)  "<pqr>"

== system Overtaking_Integrated/Vehicle Plant/Environment ==
  note: The Ground Feedback variant subsystem is automatically enabled/disabled according to the 3D Engine settings found in the Reference Generator.
      | Manually overriding this variant may result in initialization errors.
  Bus Creator1 : BusCreator  Inputs=2
  Constant3 : Constant  Value=0
  Constant4 : Constant  Value=0
  Constant5 : Constant  Value=0
  Friction : Constant  Value=ones(4,1).*1
  Ground Feedback : Subsystem  Variant=on  VariantControlMode=label  LabelModeActiveChoice=0
  Vector Concatenate : Concatenate  NumInputs=3
  Env : Outport  VectorParamsAs1DForOutWhenUnconnected=off
  wires:
  Constant5/1 -> Vector Concatenate/3  "Z"
  Vector Concatenate/1 -> Bus Creator1/1  "Wind"
  Constant3/1 -> Vector Concatenate/1  "X"
  Constant4/1 -> Vector Concatenate/2  "Y"
  Ground Feedback/1(Ground) -> Bus Creator1/2  "Gnd"
  Bus Creator1/1 -> Env/1
  Friction/1 -> Ground Feedback/1(Friction)

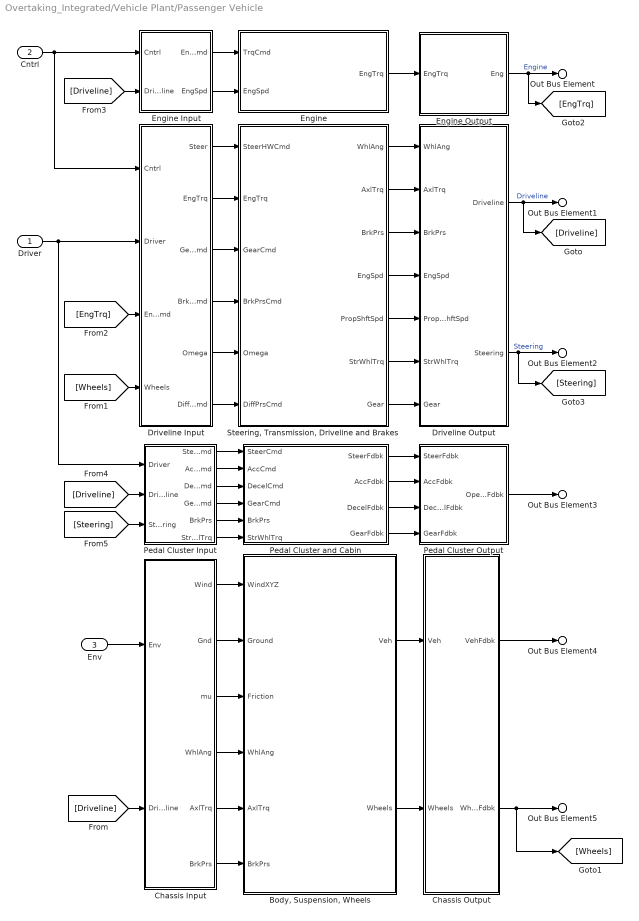
== system Overtaking_Integrated/Vehicle Plant/Passenger Vehicle ==
  Driver : Inport
  Cntrl : Inport  Port=2
  Env : Inport  Port=3
  "Body, Suspension, Wheels" : Subsystem  Variant=on  VariantControlMode=label  LabelModeActiveChoice=3
  Chassis Input : Subsystem
  Chassis Output : Subsystem
  Driveline Input : Subsystem
  Driveline Output : Subsystem
  Engine : Subsystem  Variant=on  VariantControlMode=label  LabelModeActiveChoice=0
  Engine Input : Subsystem
  Engine Output : Subsystem
  Pedal Cluster Input : Subsystem
  Pedal Cluster Output : Subsystem
  Pedal Cluster and Cabin : Subsystem
  "Steering, Transmission, Driveline and Brakes" : Subsystem  Variant=on  VariantControlMode=label  LabelModeActiveChoice=0
  Out Bus Element : Outport  PortName=VehFdbk  Element=Engine
  Out Bus Element1 : Outport  PortName=VehFdbk  Element=Driveline
  Out Bus Element2 : Outport  PortName=VehFdbk  Element=Steering
  Out Bus Element3 : Outport  PortName=VehFdbk  Element=Driver
  Out Bus Element4 : Outport  PortName=VehFdbk  Element=Body
  Out Bus Element5 : Outport  PortName=VehFdbk  Element=Wheels
  wires:
  Env/1 -> Chassis Input/1(Env)
  Chassis Input/1(Wind) -> "Body, Suspension, Wheels"/1(WindXYZ)
  Chassis Input/2(Gnd) -> "Body, Suspension, Wheels"/2(Ground)
  Chassis Input/3(mu) -> "Body, Suspension, Wheels"/3(Friction)
  Chassis Input/4(WhlAng) -> "Body, Suspension, Wheels"/4(WhlAng)
  Chassis Input/5(AxlTrq) -> "Body, Suspension, Wheels"/5(AxlTrq)
  Chassis Input/6(BrkPrs) -> "Body, Suspension, Wheels"/6(BrkPrs)
  Driveline Output/1(Driveline) -> Out Bus Element1/1, [Driveline]  "Driveline"
  "Steering, Transmission, Driveline and Brakes"/1(WhlAng) -> Driveline Output/1(WhlAng)
  "Steering, Transmission, Driveline and Brakes"/2(AxlTrq) -> Driveline Output/2(AxlTrq)
  "Steering, Transmission, Driveline and Brakes"/3(BrkPrs) -> Driveline Output/3(BrkPrs)
  "Steering, Transmission, Driveline and Brakes"/4(EngSpd) -> Driveline Output/4(EngSpd)
  "Steering, Transmission, Driveline and Brakes"/5(PropShftSpd) -> Driveline Output/5(PropShftSpd)
  Driver/1 -> Pedal Cluster Input/1(Driver), Driveline Input/2(Driver)
  Cntrl/1 -> Engine Input/1(Cntrl), Driveline Input/1(Cntrl)
  Driveline Input/1(Steer) -> "Steering, Transmission, Driveline and Brakes"/1(SteerHWCmd)
  Driveline Input/3(GearCmd) -> "Steering, Transmission, Driveline and Brakes"/3(GearCmd)
  Driveline Input/4(BrkPrsCmd) -> "Steering, Transmission, Driveline and Brakes"/4(BrkPrsCmd)
  Driveline Input/5(Omega) -> "Steering, Transmission, Driveline and Brakes"/5(Omega)
  Engine/1(EngTrq) -> Engine Output/1("EngTrq ")
  Driveline Input/2(EngTrq) -> "Steering, Transmission, Driveline and Brakes"/2(EngTrq)
  Engine Input/1(EngTrqCmd) -> Engine/1(TrqCmd)
  Engine Input/2(EngSpd) -> Engine/2(EngSpd)
  Engine Output/1(Eng) -> Out Bus Element/1, [EngTrq]  "Engine"
  [Driveline] -> Chassis Input/2(Driveline)
  [Wheels] -> Driveline Input/4(Wheels)
  [EngTrq] -> Driveline Input/3(EngTrqCmd)
  [Driveline] -> Engine Input/2(Driveline)
  Driveline Input/6(DiffPrsCmd) -> "Steering, Transmission, Driveline and Brakes"/6(DiffPrsCmd)
  "Steering, Transmission, Driveline and Brakes"/6(StrWhlTrq) -> Driveline Output/6(StrWhlTrq)
  Driveline Output/2(Steering) -> Out Bus Element2/1, [Steering]  "Steering"
  Pedal Cluster Output/1(OperatorFdbk) -> Out Bus Element3/1
  Pedal Cluster and Cabin/1(SteerFdbk) -> Pedal Cluster Output/1(SteerFdbk)
  Pedal Cluster and Cabin/2(AccFdbk) -> Pedal Cluster Output/2(AccFdbk)
  Pedal Cluster and Cabin/3(DecelFdbk) -> Pedal Cluster Output/3(DecelFdbk)
  Pedal Cluster and Cabin/4(GearFdbk) -> Pedal Cluster Output/4(GearFdbk)
  Pedal Cluster Input/4(GearCmd) -> Pedal Cluster and Cabin/4(GearCmd)
  Pedal Cluster Input/3(DecelCmd) -> Pedal Cluster and Cabin/3(DecelCmd)
  Pedal Cluster Input/2(AccelCmd) -> Pedal Cluster and Cabin/2(AccCmd)
  Pedal Cluster Input/1(SteerCmd) -> Pedal Cluster and Cabin/1(SteerCmd)
  [Driveline] -> Pedal Cluster Input/2(Driveline)
  Pedal Cluster Input/5(BrkPrs) -> Pedal Cluster and Cabin/5(BrkPrs)
  [Steering] -> Pedal Cluster Input/3(Steering)
  Pedal Cluster Input/6(StrWhlTrq) -> Pedal Cluster and Cabin/6(StrWhlTrq)
  "Body, Suspension, Wheels"/2(Wheels) -> Chassis Output/2(Wheels)
  "Body, Suspension, Wheels"/1(Veh) -> Chassis Output/1(Veh)
  Chassis Output/2(WheelsFdbk) -> [Wheels], Out Bus Element5/1
  Chassis Output/1(VehFdbk) -> Out Bus Element4/1
  "Steering, Transmission, Driveline and Brakes"/7(Gear) -> Driveline Output/7(Gear)

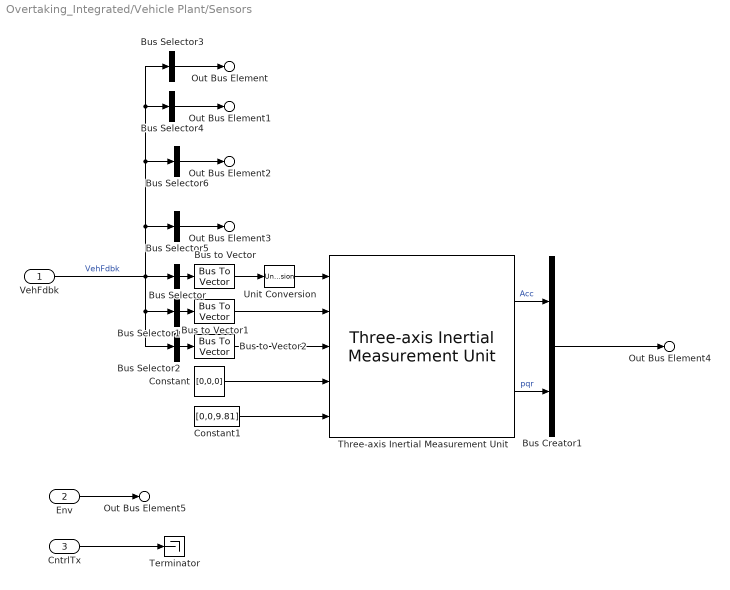
== system Overtaking_Integrated/Vehicle Plant/Sensors ==
  VehFdbk : Inport
  Env : Inport  Port=2
  CntrlTx : Inport  Port=3
  Bus Creator1 : BusCreator  Inputs=2
  Bus Selector : BusSelector  OutputSignals=Body.BdyFrm.Cg.Acc.ax,Body.BdyFrm.Cg.Acc.ay,Body.BdyFrm.Cg.Acc.az  OutputAsBus=on
  Bus Selector1 : BusSelector  OutputSignals=Body.BdyFrm.Cg.AngVel.p,Body.BdyFrm.Cg.AngVel.q,Body.BdyFrm.Cg.AngVel.r  OutputAsBus=on
  Bus Selector2 : BusSelector  OutputSignals=Body.BdyFrm.Cg.AngAcc.pdot,Body.BdyFrm.Cg.AngAcc.qdot,Body.BdyFrm.Cg.AngAcc.rdot  OutputAsBus=on
  Bus Selector3 : BusSelector  OutputSignals=Driver  OutputAsBus=on
  Bus Selector4 : BusSelector  OutputSignals=Engine.EngTrq,Driveline.EngSpd  OutputAsBus=on
  Bus Selector5 : BusSelector  OutputSignals=Driveline.BrkPrs,Wheels.TireFrame.Kappa,Wheels.TireFrame.Alpha,Wheels.TireFrame.Omega  OutputAsBus=on
  Bus Selector6 : BusSelector  OutputSignals=Driveline.PropShftSpd,Driveline.AxlTrq  OutputAsBus=on
  Bus to Vector : BusToVector
  Bus to Vector1 : BusToVector
  Bus to Vector2 : BusToVector
  Constant : Constant  Value=[0,0,0]
  Constant1 : Constant  Value=[0,0,9.81]
  Terminator : Terminator
  Three-axis Inertial Measurement Unit : vehdynlibsens/Three-axis Inertial Measurement Unit  units=Metric (MKS)  imu=[0 0 0]  i_Ts=0  dtype_a=off  w_a=190  z_a=0.707  a_sf_cc=[1 0 0; 0 1 0; 0 0 1]  a_bias=[0 0 0]  a_sat="[-inf  -inf  -inf  inf inf inf]"  dtype_g=off  w_g=190  z_g=0.707  g_sf_cc=[1 0 0; 0 1 0; 0 0 1]  g_bias=[0 0 0]  g_sens=[0 0 0]  g_sat="[-inf  -inf  -inf  inf inf inf]"  i_rand=on  i_seeds=[23093 23094 23095 23096 23097 23098]  i_pow=[0.001 0.001 0.001 0.0001 0.0001 0.0001]  aMode=2
      settings: SourceProductBaseCode=VE
  Unit Conversion : UnitConversion
  Out Bus Element : Outport  PortName=CntrlRx  Element=Driver
  Out Bus Element1 : Outport  PortName=CntrlRx  Element=Engine
  Out Bus Element2 : Outport  PortName=CntrlRx  Element=Trans
  Out Bus Element3 : Outport  PortName=CntrlRx  Element=Wheels
  Out Bus Element4 : Outport  PortName=CntrlRx  Element=IMU
  Out Bus Element5 : Outport  PortName=CntrlRx  Element=Env
  wires:
  VehFdbk/1 -> Bus Selector/1, Bus Selector2/1, Bus Selector1/1, Bus Selector6/1, Bus Selector3/1, Bus Selector4/1, Bus Selector5/1  "VehFdbk"
  Bus Creator1/1 -> Out Bus Element4/1
  Three-axis Inertial Measurement Unit/1 -> Bus Creator1/1  "Acc"
  Three-axis Inertial Measurement Unit/2 -> Bus Creator1/2  "pqr"
  Bus Selector/1 -> Bus to Vector/1
  Bus to Vector/1 -> Unit Conversion/1
  Bus Selector1/1 -> Bus to Vector1/1
  Bus to Vector1/1 -> Three-axis Inertial Measurement Unit/2
  Env/1 -> Out Bus Element5/1
  Bus Selector2/1 -> Bus to Vector2/1
  Bus to Vector2/1 -> Three-axis Inertial Measurement Unit/3
  Constant/1 -> Three-axis Inertial Measurement Unit/4
  Constant1/1 -> Three-axis Inertial Measurement Unit/5
  Unit Conversion/1 -> Three-axis Inertial Measurement Unit/1
  CntrlTx/1 -> Terminator/1
  Bus Selector3/1 -> Out Bus Element/1
  Bus Selector4/1 -> Out Bus Element1/1
  Bus Selector5/1 -> Out Bus Element3/1
  Bus Selector6/1 -> Out Bus Element2/1

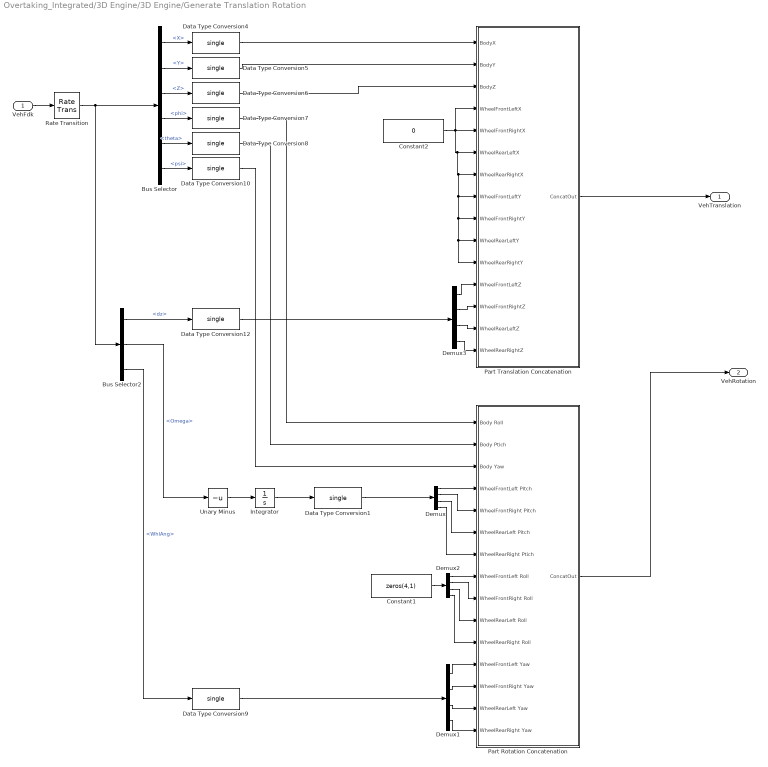
== system Overtaking_Integrated/3D Engine/3D Engine/Generate Translation Rotation ==
  VehFdk : Inport
  Bus Selector : BusSelector  OutputSignals=Body.InertFrm.Geom.Disp.X,Body.InertFrm.Geom.Disp.Y,Body.InertFrm.Geom.Disp.Z,Body.InertFrm.Cg.Ang.phi,Body.InertFrm.Cg.Ang.theta,Body.InertFrm.Cg.Ang.psi
  Bus Selector2 : BusSelector  OutputSignals=Wheels.TireFrame.dz,Wheels.TireFrame.Omega,Driveline.WhlAng
  Constant1 : Constant  Value=zeros(4,1)  OutDataTypeStr=single
  Constant2 : Constant  Value=0  OutDataTypeStr=single
  Data Type Conversion{1,4..10,12} (9 alike) : DataTypeConversion  OutDataTypeStr=single
  Demux{,1..3} (4 alike) : Demux
  Integrator : Integrator  WrapState=on  WrappedStateUpperValue=2*pi  WrappedStateLowerValue=0  ZeroCross=off
  Part Rotation Concatenation : Subsystem
  Part Translation Concatenation : Subsystem
  Rate Transition : RateTransition  OutPortSampleTime=dt3D
  Unary Minus : UnaryMinus
  VehTranslation : Outport
  VehRotation : Outport  Port=2
  wires:
  Demux/3 -> Part Rotation Concatenation/6(WheelRearLeft Pitch)
  Integrator/1 -> Data Type Conversion1/1
  Demux1/4 -> Part Rotation Concatenation/15(WheelRearRight Yaw)
  Constant2/1 -> Part Translation Concatenation/5(WheelFrontRightX), Part Translation Concatenation/6(WheelRearLeftX), Part Translation Concatenation/7(WheelRearRightX), Part Translation Concatenation/8(WheelFrontLeftY), Part Translation Concatenation/9(WheelFrontRightY), Part Translation Concatenation/10(WheelRearLeftY), Part Translation Concatenation/11(WheelRearRightY), Part Translation Concatenation/4(WheelFrontLeftX)
  Demux3/4 -> Part Translation Concatenation/15(WheelRearRightZ)
  Rate Transition/1 -> Bus Selector/1, Bus Selector2/1
  Unary Minus/1 -> Integrator/1
  Constant1/1 -> Demux2/1
  Demux/4 -> Part Rotation Concatenation/7(WheelRearRight Ptich)
  Data Type Conversion12/1 -> Demux3/1
  Bus Selector2/1 -> Data Type Conversion12/1  "<dz>"
  Data Type Conversion6/1 -> Part Translation Concatenation/3(BodyZ)
  Data Type Conversion9/1 -> Demux1/1
  Demux/2 -> Part Rotation Concatenation/5(WheelFrontRight Pitch)
  Demux/1 -> Part Rotation Concatenation/4(WheelFrontLeft Pitch)
  Demux2/2 -> Part Rotation Concatenation/9(WheelFrontRight Roll)
  Demux2/4 -> Part Rotation Concatenation/11(WheelRearRight Roll)
  Demux3/1 -> Part Translation Concatenation/12(WheelFrontLeftZ)
  Demux3/3 -> Part Translation Concatenation/14(WheelRearLeftZ)
  Bus Selector/2 -> Data Type Conversion5/1  "<Y>"
  Part Rotation Concatenation/1(ConcatOut) -> VehRotation/1
  Demux2/3 -> Part Rotation Concatenation/10(WheelRearLeft Roll)
  Data Type Conversion5/1 -> Part Translation Concatenation/2(BodyY)
  Data Type Conversion4/1 -> Part Translation Concatenation/1(BodyX)
  Data Type Conversion7/1 -> Part Rotation Concatenation/1(Body Roll)
  Data Type Conversion8/1 -> Part Rotation Concatenation/2(Body Ptich)
  Bus Selector2/3 -> Data Type Conversion9/1  "<WhlAng>"
  Demux1/3 -> Part Rotation Concatenation/14(WheelRearLeft Yaw)
  Data Type Conversion10/1 -> Part Rotation Concatenation/3(Body Yaw)
  Data Type Conversion1/1 -> Demux/1
  Bus Selector/1 -> Data Type Conversion4/1  "<X>"
  Bus Selector/3 -> Data Type Conversion6/1  "<Z>"
  Bus Selector/6 -> Data Type Conversion10/1  "<psi>"
  Demux1/2 -> Part Rotation Concatenation/13(WheelFrontRight Yaw)
  VehFdk/1 -> Rate Transition/1
  Demux1/1 -> Part Rotation Concatenation/12(WheelFrontLeft Yaw)
  Bus Selector2/2 -> Unary Minus/1  "<Omega>"
  Demux2/1 -> Part Rotation Concatenation/8(WheelFrontLeft Roll)
  Demux3/2 -> Part Translation Concatenation/13(WheelFrontRightZ)
  Bus Selector/4 -> Data Type Conversion7/1  "<phi>"
  Bus Selector/5 -> Data Type Conversion8/1  "<theta>"
  Part Translation Concatenation/1(ConcatOut) -> VehTranslation/1

== system Overtaking_Integrated/3D Engine/3D Engine/Scale ==
  Constant{1..12,17,32..33} (15 alike) : Constant  OutDataTypeStr=single
  PartConcatenation : Subsystem
  ScaleOut : Outport  VectorParamsAs1DForOutWhenUnconnected=off
  wires:
  Constant10/1 -> PartConcatenation/15(WheelRearRightZ)
  Constant9/1 -> PartConcatenation/14(WheelRearRightY)
  Constant11/1 -> PartConcatenation/13(WheelRearRightX)
  Constant7/1 -> PartConcatenation/12(WheelRearLeftZ)
  Constant6/1 -> PartConcatenation/11(WheelRearLeftY)
  Constant8/1 -> PartConcatenation/10(WheelRearLeftX)
  Constant4/1 -> PartConcatenation/9(WheelFrontRightZ)
  Constant3/1 -> PartConcatenation/8(WheelFrontRightY)
  Constant5/1 -> PartConcatenation/7(WheelFrontRightX)
  Constant2/1 -> PartConcatenation/6(WheelFrontLeftZ)
  Constant1/1 -> PartConcatenation/5(WheelFrontLeftY)
  Constant33/1 -> PartConcatenation/4(WheelFrontLeftX)
  Constant32/1 -> PartConcatenation/3(BodyZ)
  Constant17/1 -> PartConcatenation/2(BodyY)
  Constant12/1 -> PartConcatenation/1(BodyX)
  PartConcatenation/1(ConcatOut) -> ScaleOut/1

== system Overtaking_Integrated/ScenarioSetup/Scenario Reader/SAE J670E to ISO 8855 (NED to NWU) ==
  note: SAE J670E to ISO 8855
  Position : Inport  Unit=m
  Velocity : Inport  Port=2  Unit=m/s
  Yaw Angle : Inport  Port=3  Unit=deg
  Yaw Rate : Inport  Port=4  Unit=deg/s
  Demux : Demux  Outputs=2
  Demux1 : Demux  Outputs=2
  Mux : Mux  Inputs=2
  Mux1 : Mux  Inputs=2
  Unary Minus{,1..3} (4 alike) : UnaryMinus
  1 : Outport  VectorParamsAs1DForOutWhenUnconnected=off
  2 : Outport  Port=2  VectorParamsAs1DForOutWhenUnconnected=off
  3 : Outport  Port=3  VectorParamsAs1DForOutWhenUnconnected=off
  4 : Outport  Port=4  VectorParamsAs1DForOutWhenUnconnected=off
  wires:
  Yaw Rate/1 -> Unary Minus3/1
  Yaw Angle/1 -> Unary Minus2/1
  Demux/1 -> Mux/1
  Demux/2 -> Unary Minus/1
  Unary Minus/1 -> Mux/2
  Unary Minus1/1 -> Mux1/2
  Demux1/2 -> Unary Minus1/1
  Demux1/1 -> Mux1/1
  Mux1/1 -> 2/1
  Mux/1 -> 1/1
  Position/1 -> Demux/1
  Velocity/1 -> Demux1/1
  Unary Minus2/1 -> 3/1
  Unary Minus3/1 -> 4/1
